simulink model "simulink_experiments_LQ_der_SwingUp"  (R2019b)
settings: Solver=ode1  StartTime=0.0  StopTime=inf  FixedStep=0.002  RelTol=1e-3  EnableMultiTasking=on
PostLoadFcn:
  | qc_set_target_type(getConfigSet(bdroot, 'QUARC Default Target Configuration'));
undefined symbols (not defined in the file): HIL, Klqi_int, Klqi_state, Kpp_int, Kpp_state, Parameters, qc_get_step_size
libraries: quarc_library x4
settings Model: SimulationMode=external  ExtModeTrigDuration=5000  Creator=CFulford  LastModifiedBy=pietr
settings SolverCC: PositivePriorityOrder=on
settings DataIOCC: LimitDataPoints=on  SaveFormat=Array  SignalLoggingSaveFormat=ModelDataLogs  ReturnWorkspaceOutputs=off
settings OptimizationCC: ExpressionDepthLimit=2147483647  InitFltsAndDblsToZero=on  LifeSpan=inf
settings DebuggingCC: SaveWithParameterizedLinksMsg=none  UnderspecifiedInitializationDetection=Classic  MergeDetectMultiDrivingBlocksExec=none  SolverPrmCheckMsg=warning  MultiTaskDSMMsg=warning  MultiTaskCondExecSysMsg=none  FcnCallInpInsideContextMsg=warning  StateNameClashWarn=warning  SFUnexpectedBacktrackingDiag=warning  SFNoUnconditionalDefaultTransitionDiag=warning  SFExecutionAtInitializationDiag=none  ArithmeticOperatorsInVariantConditions=warning
settings HardwareCC: ProdBitPerPointer=32  ProdBitPerSizeT=32  ProdBitPerPtrDiffT=32  ProdLargestAtomicFloat=None  ProdIntDivRoundTo=Undefined  ProdEndianess=Unspecified  ProdWordSize=32  ProdHWDeviceType=32-bit Generic
settings ModelReferenceCC: PropagateSignalLabelsOutOfModel=off
settings SFSimCC: SimUseLocalCustomCode=off  CustomCodeUndefinedFunction=UseInterfaceOnly
settings RTWCC: Description=QUARC Win64 Target  SystemTargetFile=quarc_win64.tlc  TemplateMakefile=quarc_default_tmf  RTWUseLocalCustomCode=off
settings CodeAppCC: StateflowObjectComments=on
settings STFCustomTargetCC: TargetPreCompLibLocation=C:\PROGRA~3\QUARC\lib\2019b\win64\release  ConcurrentExecutionCompliant=on  GeneratePreprocessorConditionals=Disable all  CombineOutputUpdateFcns=on  CPPClassGenCompliant=on  SystemTargetFile=quarc_win64.tlc
settings GRTTargetCC: TargetPreCompLibLocation=C:\PROGRA~3\QUARC\lib\2019b\win64\release  TargetLangStandard=C89/C90 (ANSI)  ParMdlRefBuildCompliant=off  CompOptLevelCompliant=off  GeneratePreprocessorConditionals=Disable all  MatFileLogging=off  UseToolchainInfoCompliant=off  ExtMode=on  ExtModeMexFile=quarc_comm
settings ConfigComp: CovMetricSettings=dw  CovHtmlReporting=on  CovSaveCumulativeToWorkspaceVar=on  CovSaveSingleToWorkspaceVar=on  CovExternalEMLEnable=off  CovSFcnEnable=off

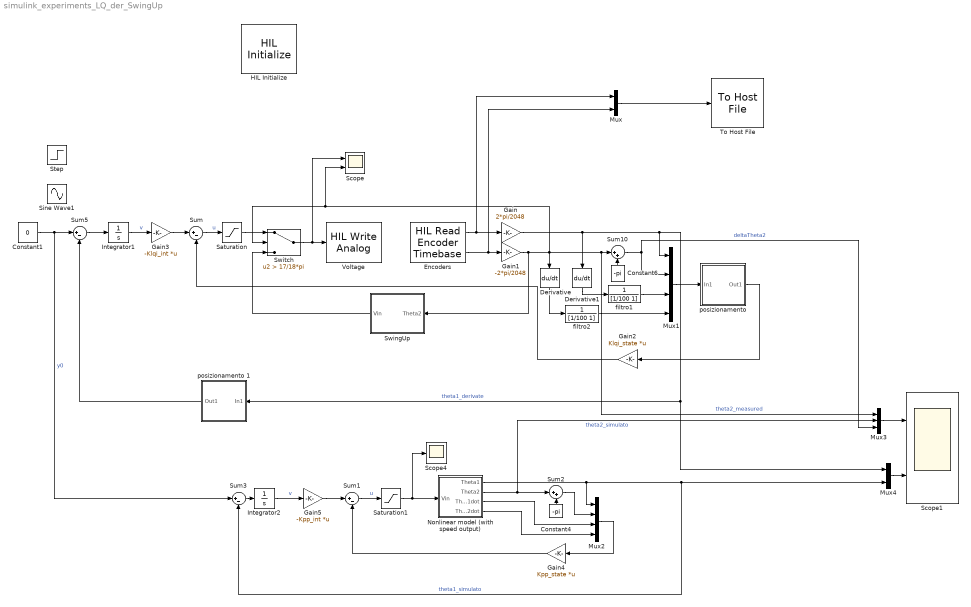
== system simulink_experiments_LQ_der_SwingUp ==
  Constant1 : Constant  Value=0
  Constant4 : Constant  Value=-pi
  Constant6 : Constant  Value=-pi
  Derivative : Derivative
  Derivative1 : Derivative
  Encoders : quarc_library/Data Acquisition/Generic/Timebases/HIL Read Encoder Timebase  object_name=HIL-1  clock=0  channels=[0:1]  samples_in_buffer=max(ceil(1/qc_get_step_size), 1)  active=on  vector_output=off  data_type_mode=Inherit via back propagation  data_type=double
  Gain : Gain  Gain=2*pi/2048
  Gain1 : Gain  Gain=-2*pi/2048
  Gain2 : Gain  Gain=Klqi_state  Multiplication=Matrix(K*u)
  Gain3 : Gain  Gain=-Klqi_int  Multiplication=Matrix(K*u)
  Gain4 : Gain  Gain=Kpp_state  Multiplication=Matrix(K*u)
  Gain5 : Gain  Gain=-Kpp_int  Multiplication=Matrix(K*u)
  HIL Initialize : quarc_library/Data Acquisition/Generic/Configuration/HIL Initialize  Priority=-99  object_name=HIL-1  board_type=qube_servo2_usb  board_number=0  board_options=""  exclusive=off  active=off  hardware_clocks=[0]  clock_modes=[]  initial_clock_frequencies=[]  set_clock_params_at_start=off  set_clock_params_at_switch_in=off  set_clock_frequencies_at_start=off  set_clock_frequencies_at_switch_in=off  analog_input_channels=[0]  analog_input_configurations=[]  analog_input_maximums=3  analog_input_minimums=-3  set_analog_input_params_at_start=off  set_analog_input_params_at_switch_in=off  analog_output_channels=[0]  analog_output_maximums=15  analog_output_minimums=-15  initial_analog_outputs=[0]  final_analog_outputs=[0]  watchdog_analog_outputs=0  set_analog_output_params_at_start=off  set_analog_output_params_at_switch_in=off  set_analog_outputs_at_start=on  set_analog_outputs_at_switch_in=off  set_analog_outputs_at_terminate=on  set_analog_outputs_at_switch_out=off  set_analog_outputs_on_watchdog=on  digital_input_channels=[]  digital_output_channels=[0]  digital_output_configuration=[]  initial_digital_outputs=[1]  final_digital_outputs=[0]  watchdog_digital_outputs=[0]  set_digital_output_params_at_start=off  set_digital_output_params_at_switch_in=off  set_digital_outputs_at_start=on  set_digital_outputs_at_switch_in=off  set_digital_outputs_at_terminate=on  set_digital_outputs_at_switch_out=off  set_digital_outputs_on_watchdog=on  encoder_channels=[0:1]  quadrature=[4]  encoder_filter_frequency=[]  initial_encoder_counts=[0]  set_encoder_params_at_start=off  set_encoder_params_at_switch_in=off  set_encoder_counts_at_start=on  set_encoder_counts_at_switch_in=off  pwm_channels=[]  pwm_modes=[]  pwm_frequency=[]  pwm_configuration=[]  pwm_alignment=[]  pwm_polarity=[]  pwm_leading_deadband=[]  pwm_trailing_deadband=[]  initial_pwm_outputs=[]  final_pwm_outputs=[]  watchdog_pwm_outputs=[]  set_pwm_params_at_start=off  set_pwm_params_at_switch_in=off  set_pwm_outputs_at_start=off  set_pwm_outputs_at_switch_in=off  set_pwm_outputs_at_terminate=off  set_pwm_outputs_at_switch_out=off  set_pwm_outputs_on_watchdog=off  other_output_channels=[11000:11002]  initial_other_outputs=[0 1 0]  final_other_outputs=[1 0 0]  watchdog_other_outputs=[0 0 1]  set_other_outputs_at_start=on  set_other_outputs_at_switch_in=off  set_other_outputs_at_terminate=on  set_other_outputs_at_switch_out=off  set_other_outputs_on_watchdog=on
  Integrator1 : Integrator
  Integrator2 : Integrator
  Mux : Mux  Inputs=2
  Mux1 : Mux
  Mux2 : Mux
  Mux3 : Mux  Inputs=3
  Mux4 : Mux  Inputs=2
  Nonlinear model (with speed output) : Subsystem
  Saturation : Saturate  UpperLimit=10  LowerLimit=-10
  Saturation1 : Saturate  UpperLimit=10  LowerLimit=-10
  Scope : Scope  NumInputPorts=2
  Scope1 : Scope  NumInputPorts=2
  Scope4 : Scope
  Sine Wave1 : Sin  SampleTime=0
  Step : Step  Time=10  SampleTime=0
  Sum{,1,3,5} (4 alike) : Sum  Inputs=|+-
  Sum10 : Sum  Inputs=|++
  Sum2 : Sum  Inputs=|++
  SwingUp : Subsystem
  Switch : Switch  Criteria=u2 > Threshold  Threshold=17/18*pi
  To Host File : quarc_library/Sinks/To Host/To Host File  file_name=data_%{date}_%{time}.mat  variable_name=data_%{date}_%{time}  decimation=1  sample_time=-1  file_format=MAT-file v.5  options=No header or footer  append=off  final_file_name=data_07-May-2024_17-23-06.mat  bitrate=2000000
  Voltage : quarc_library/Data Acquisition/Generic/Immediate I//O/HIL Write Analog  object_name=HIL-1  channels=0  sample_time=-1  active=off  vector_input=off
  "filtro1 " : TransferFcn  Denominator=[1/100 1]
  filtro2 : TransferFcn  Denominator=[1/100 1]
  "posizionamento " : Subsystem
  posizionamento 1 : Subsystem
  wires:
  Nonlinear model (with speed output)/1(Theta1) -> Mux4/2, Sum3/2, Mux2/1  "theta1_simulato"
  posizionamento 1/1(Out1) -> Sum5/2
  Nonlinear model (with speed output)/4(Theta2dot) -> Mux2/4
  Mux1/1 -> "posizionamento "/1(In1)
  "posizionamento "/1(Out1) -> Gain2/1
  Gain/1 -> Mux4/1, posizionamento 1/1(In1), Mux1/1, Derivative1/1  "theta1_derivate"
  Mux3/1 -> Scope1/1
  Constant4/1 -> Sum2/2
  Constant6/1 -> Sum10/2
  Sum2/1 -> Mux2/2
  Mux/1 -> To Host File/1
  Nonlinear model (with speed output)/2(Theta2) -> Mux3/2, Sum2/1  "theta2_simulato"
  Sum3/1 -> Integrator2/1
  Sum1/1 -> Saturation1/1  "u"
  Nonlinear model (with speed output)/3(Theta1dot) -> Mux2/3
  Mux2/1 -> Gain4/1
  Derivative1/1 -> "filtro1 "/1
  Gain5/1 -> Sum1/1
  Gain4/1 -> Sum1/2
  Mux4/1 -> Scope1/2
  "filtro1 "/1 -> Mux1/3
  filtro2/1 -> Mux1/4
  Saturation1/1 -> Nonlinear model (with speed output)/1(Vin), Scope4/1
  Encoders/1 -> Gain/1, Mux/1
  Integrator2/1 -> Gain5/1  "v"
  Gain3/1 -> Sum/1
  Gain2/1 -> Sum/2
  Sum/1 -> Saturation/1  "u"
  Gain1/1 -> SwingUp/1(Theta2), Scope/2, Switch/2, Mux3/1, Sum10/1, Derivative/1  "theta2_measured"
  Sum5/1 -> Integrator1/1
  Constant1/1 -> Sum3/1, Sum5/1  "y0"
  Integrator1/1 -> Gain3/1  "v"
  Derivative/1 -> filtro2/1
  Encoders/2 -> Gain1/1, Mux/2
  Sum10/1 -> Mux1/2, Mux3/3  "deltaTheta2"
  Saturation/1 -> Switch/1
  Switch/1 -> Scope/1, Voltage/1
  SwingUp/1(Vin) -> Switch/3

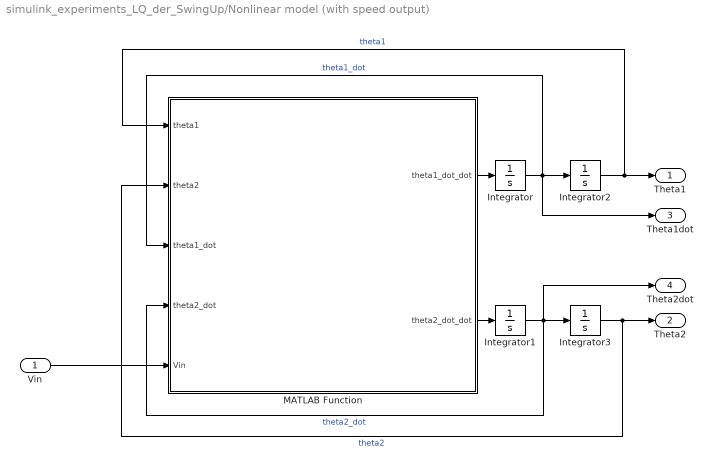
== system simulink_experiments_LQ_der_SwingUp/Nonlinear model (with speed output) ==
  Vin : Inport
  Integrator : Integrator
  Integrator1 : Integrator
  Integrator2 : Integrator
  Integrator3 : Integrator  InitialCondition=pi+0.3
  MATLAB Function : MATLAB Function  TreatAsAtomicUnit=on  mask{Pars=Parameters}
      mask prompts: Pars "Struct containing model parameters"
  Theta1 : Outport
  Theta2 : Outport  Port=2
  Theta1dot : Outport  Port=3
  Theta2dot : Outport  Port=4
  wires:
  Integrator/1 -> Theta1dot/1, MATLAB Function/3(theta1_dot), Integrator2/1  "theta1_dot"
  Integrator1/1 -> Theta2dot/1, MATLAB Function/4(theta2_dot), Integrator3/1  "theta2_dot"
  MATLAB Function/1(theta1_dot_dot) -> Integrator/1
  Integrator3/1 -> Theta2/1, MATLAB Function/2(theta2)  "theta2"
  MATLAB Function/2(theta2_dot_dot) -> Integrator1/1
  Integrator2/1 -> MATLAB Function/1(theta1), Theta1/1  "theta1"
  Vin/1 -> MATLAB Function/5(Vin)

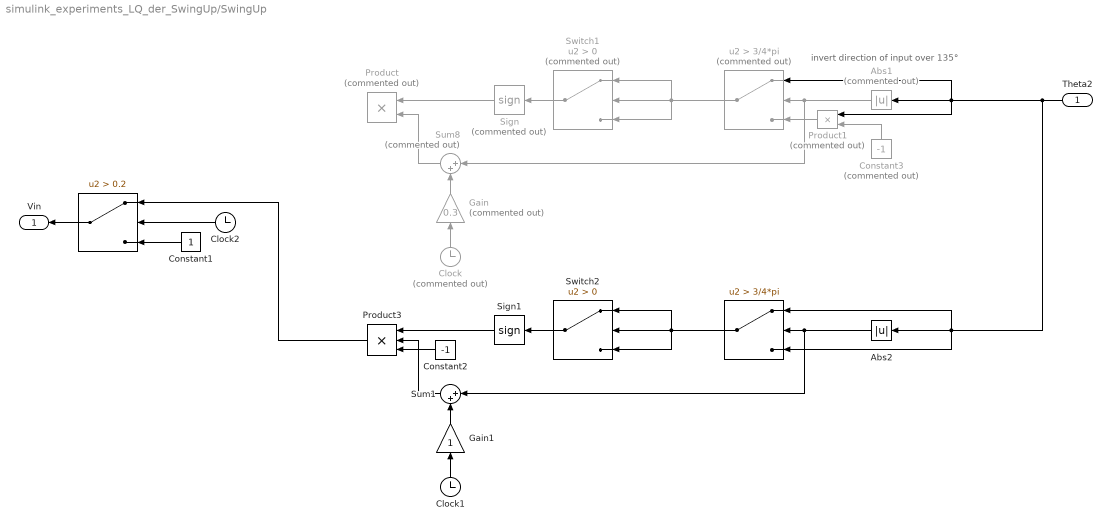
== system simulink_experiments_LQ_der_SwingUp/SwingUp ==
  note: invert direction of input over 135°
  Theta2 : Inport
  " " : Switch  Commented=on  Criteria=u2 > Threshold  Threshold=3/4*pi
  " " : Switch  Criteria=u2 > Threshold  Threshold=3/4*pi
  " " : Switch  Criteria=u2 > Threshold  Threshold=0.2
  Abs1 : Abs  Commented=on
  Abs2 : Abs
  Clock : Clock  Commented=on
  Clock1 : Clock
  Clock2 : Clock
  Constant1 : Constant
  Constant2 : Constant  Value=-1
  Constant3 : Constant  Commented=on  Value=-1
  Gain : Gain  Commented=on  Gain=0.3
  Gain1 : Gain
  Product : Product  Commented=on
  Product1 : Product  Commented=on
  Product3 : Product  Inputs=3
  Sign : Signum  Commented=on
  Sign1 : Signum
  Sum1 : Sum  Inputs=|++
  Sum8 : Sum  Commented=on  Inputs=|++
  Switch1 : Switch  Commented=on  Criteria=u2 > Threshold
  Switch2 : Switch  Criteria=u2 > Threshold
  Vin : Outport
  wires:
  Abs1/1 -> Sum8/1, " "/2
  " "/1 -> Switch1/3, Switch1/2, Switch1/1
  Constant3/1 -> Product1/2
  Clock/1 -> Gain/1
  Product1/1 -> " "/3
  Switch1/1 -> Sign/1
  Gain/1 -> Sum8/2
  Sign/1 -> Product/1
  Sum8/1 -> Product/2
  Sign1/1 -> Product3/1
  Sum1/1 -> Product3/2
  Switch2/1 -> Sign1/1
  " "/1 -> Switch2/3, Switch2/2, Switch2/1
  Clock1/1 -> Gain1/1
  Gain1/1 -> Sum1/2
  Theta2/1 -> " "/1, " "/3, Abs2/1, Product1/1, Abs1/1, " "/1
  Abs2/1 -> Sum1/1, " "/2
  Constant2/1 -> Product3/3
  Clock2/1 -> " "/2
  Constant1/1 -> " "/3
  " "/1 -> Vin/1
  Product3/1 -> " "/1

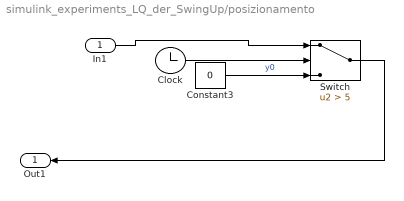
== system simulink_experiments_LQ_der_SwingUp/posizionamento  ==
  In1 : Inport
  Clock : Clock
  Constant3 : Constant  Value=0
  Switch : Switch  Criteria=u2 > Threshold  Threshold=5
  Out1 : Outport
  wires:
  In1/1 -> Switch/1
  Constant3/1 -> Switch/3  "y0"
  Clock/1 -> Switch/2
  Switch/1 -> Out1/1

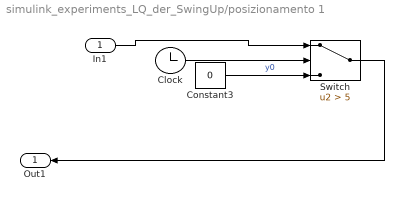
== system simulink_experiments_LQ_der_SwingUp/posizionamento 1 ==
  In1 : Inport
  Clock : Clock
  Constant3 : Constant  Value=0
  Switch : Switch  Criteria=u2 > Threshold  Threshold=5
  Out1 : Outport
  wires:
  In1/1 -> Switch/1
  Constant3/1 -> Switch/3  "y0"
  Clock/1 -> Switch/2
  Switch/1 -> Out1/1

== matlab function simulink_experiments_LQ_der_SwingUp/Nonlinear model (with speed output)/MATLAB Function ==
  data: theta1 input; theta1_dot_dot output; theta2 input; theta1_dot input; theta2_dot input; Vin input; theta2_dot_dot output; Pars parameter
function [theta1_dot_dot,theta2_dot_dot] = fcn(theta1, theta2, theta1_dot, theta2_dot,Vin, Pars)

   k1 = Pars.Jeq + Pars.m2*(Pars.l1^2 + Pars.x2^2*sin(theta2)^2);
   k2 = Pars.m2*Pars.l1*Pars.x2*cos(theta2);
   k3 = 2*Pars.m2*Pars.x2^2*sin(theta2)*cos(theta2)*theta1_dot*theta2_dot - Pars.m2*Pars.l1*Pars.x2*sin(theta2)*theta2_dot^2 +Pars.Ks*theta1 - Pars.Km/Pars.Rm*Vin + (Pars.Km^2)/Pars.Rm*theta1_dot + Pars.Kf1*theta1_dot;
   k4 = Pars.m2*Pars.l1*Pars.x2*cos(theta2);
   k5 = Pars.m2*Pars.x2^2 + Pars.I2;
   k6 = - Pars.m2*Pars.x2^2*sin(theta2)*cos(theta2)*theta1_dot^2 + Pars.m2*Pars.g*Pars.x2*sin(theta2) + Pars.Kf2*theta2_dot;


theta1_dot_dot = (k2*k6 - k3*k5)/(k1*k5 - k2*k4);
theta2_dot_dot = -(k1*k6 - k3*k4)/(k1*k5 - k2*k4);
